simulink model "c00020M_harness"  (R2018a)
settings: Solver=ode3  StartTime=0.0  StopTime=10.0  RelTol=1e-3  EnableMultiTasking=on
undefined symbols (not defined in the file): b, DiscIntNeverNeededParam, J, K, L, PosMinimaW4, R, sigbuilder_block
(part 6 of 41)

== system c00020M_harness/M020 ==
  DW1 : Inport  OutMin=0  OutMax=4  OutDataTypeStr=int8
  DW4 : Inport  Port=2  OutMin=0  OutMax=4  OutDataTypeStr=int8
  P1W2 : Inport  Port=3  OutMin=0  OutMax=4  OutDataTypeStr=int8
  P3W4 : Inport  Port=4  OutMin=0  OutMax=4  OutDataTypeStr=int8
  O1 : Inport  Port=5  OutDataTypeStr=boolean
  O2 : Inport  Port=6  OutDataTypeStr=boolean
  O4 : Inport  Port=7  OutDataTypeStr=boolean
  LD : Inport  Port=8  OutDataTypeStr=boolean
  Cyber : Subsystem
  M : Memory
  M1 : Memory
  M3 : Memory
  Physical : Subsystem
  S1 : Subsystem
  S2 : Subsystem
  S4 : Subsystem
  W1Pos : Outport
  W2Pos : Outport  Port=2
  W4Pos : Outport  Port=3
  wires:
  Cyber/3(W4) -> Physical/3(InW4)
  DW4/1 -> Cyber/5(DW4)
  Physical/3(W4) -> S4/1(PhyMeasure), W4Pos/1
  P3W4/1 -> Cyber/7(P3W4)
  S2/1(SensorOut) -> M1/1
  Physical/2(W2) -> S2/1(PhyMeasure), W2Pos/1
  DW1/1 -> Cyber/4(DW1)
  M/1 -> Cyber/1(PosW1)
  M1/1 -> Cyber/2(PosW2)
  S4/1(SensorOut) -> M3/1
  P1W2/1 -> Cyber/6(P1W2)
  Cyber/2(W2) -> Physical/2(InW2)
  Cyber/1(W1) -> Physical/1(InW1)
  O1/1 -> Cyber/8(OW1)
  LD/1 -> Cyber/11(LD)
  O2/1 -> Cyber/9(OW2)
  O4/1 -> Cyber/10(OW4)
  Physical/1(W1) -> S1/1(PhyMeasure), W1Pos/1
  S1/1(SensorOut) -> M/1
  M3/1 -> Cyber/3(PosW4)

== system c00020M_harness/M022 ==
  DW1 : Inport  OutMin=0  OutMax=4  OutDataTypeStr=int8
  DW4 : Inport  Port=2  OutMin=0  OutMax=4  OutDataTypeStr=int8
  P1W2 : Inport  Port=3  OutMin=0  OutMax=4  OutDataTypeStr=int8
  P3W4 : Inport  Port=4  OutMin=0  OutMax=4  OutDataTypeStr=int8
  O1 : Inport  Port=5  OutDataTypeStr=boolean
  O2 : Inport  Port=6  OutDataTypeStr=boolean
  O4 : Inport  Port=7  OutDataTypeStr=boolean
  LD : Inport  Port=8  OutDataTypeStr=boolean
  Cyber : Subsystem
  M : Memory
  M1 : Memory
  M3 : Memory
  Physical : Subsystem
  S1 : Subsystem
  S2 : Subsystem
  S4 : Subsystem
  W1Pos : Outport
  W2Pos : Outport  Port=2
  W4Pos : Outport  Port=3
  wires:
  Cyber/3(W4) -> Physical/3(InW4)
  DW4/1 -> Cyber/5(DW4)
  Physical/3(W4) -> S4/1(PhyMeasure), W4Pos/1
  P3W4/1 -> Cyber/7(P3W4)
  S2/1(SensorOut) -> M1/1
  Physical/2(W2) -> S2/1(PhyMeasure), W2Pos/1
  DW1/1 -> Cyber/4(DW1)
  M/1 -> Cyber/1(PosW1)
  M1/1 -> Cyber/2(PosW2)
  S4/1(SensorOut) -> M3/1
  P1W2/1 -> Cyber/6(P1W2)
  Cyber/2(W2) -> Physical/2(InW2)
  Cyber/1(W1) -> Physical/1(InW1)
  O1/1 -> Cyber/8(OW1)
  LD/1 -> Cyber/11(LD)
  O2/1 -> Cyber/9(OW2)
  O4/1 -> Cyber/10(OW4)
  Physical/1(W1) -> S1/1(PhyMeasure), W1Pos/1
  S1/1(SensorOut) -> M/1
  M3/1 -> Cyber/3(PosW4)

== system c00020M_harness/M023 ==
  DW1 : Inport  OutMin=0  OutMax=4  OutDataTypeStr=int8
  DW4 : Inport  Port=2  OutMin=0  OutMax=4  OutDataTypeStr=int8
  P1W2 : Inport  Port=3  OutMin=0  OutMax=4  OutDataTypeStr=int8
  P3W4 : Inport  Port=4  OutMin=0  OutMax=4  OutDataTypeStr=int8
  O1 : Inport  Port=5  OutDataTypeStr=boolean
  O2 : Inport  Port=6  OutDataTypeStr=boolean
  O4 : Inport  Port=7  OutDataTypeStr=boolean
  LD : Inport  Port=8  OutDataTypeStr=boolean
  Cyber : Subsystem
  M : Memory
  M1 : Memory
  M3 : Memory
  Physical : Subsystem
  S1 : Subsystem
  S2 : Subsystem
  S4 : Subsystem
  W1Pos : Outport
  W2Pos : Outport  Port=2
  W4Pos : Outport  Port=3
  wires:
  Cyber/3(W4) -> Physical/3(InW4)
  DW4/1 -> Cyber/5(DW4)
  Physical/3(W4) -> S4/1(PhyMeasure), W4Pos/1
  P3W4/1 -> Cyber/7(P3W4)
  S2/1(SensorOut) -> M1/1
  Physical/2(W2) -> S2/1(PhyMeasure), W2Pos/1
  DW1/1 -> Cyber/4(DW1)
  M/1 -> Cyber/1(PosW1)
  M1/1 -> Cyber/2(PosW2)
  S4/1(SensorOut) -> M3/1
  P1W2/1 -> Cyber/6(P1W2)
  Cyber/2(W2) -> Physical/2(InW2)
  Cyber/1(W1) -> Physical/1(InW1)
  O1/1 -> Cyber/8(OW1)
  LD/1 -> Cyber/11(LD)
  O2/1 -> Cyber/9(OW2)
  O4/1 -> Cyber/10(OW4)
  Physical/1(W1) -> S1/1(PhyMeasure), W1Pos/1
  S1/1(SensorOut) -> M/1
  M3/1 -> Cyber/3(PosW4)

== system c00020M_harness/M024 ==
  DW1 : Inport  OutMin=0  OutMax=4  OutDataTypeStr=int8
  DW4 : Inport  Port=2  OutMin=0  OutMax=4  OutDataTypeStr=int8
  P1W2 : Inport  Port=3  OutMin=0  OutMax=4  OutDataTypeStr=int8
  P3W4 : Inport  Port=4  OutMin=0  OutMax=4  OutDataTypeStr=int8
  O1 : Inport  Port=5  OutDataTypeStr=boolean
  O2 : Inport  Port=6  OutDataTypeStr=boolean
  O4 : Inport  Port=7  OutDataTypeStr=boolean
  LD : Inport  Port=8  OutDataTypeStr=boolean
  Cyber : Subsystem
  M : Memory
  M1 : Memory
  M3 : Memory
  Physical : Subsystem
  S1 : Subsystem
  S2 : Subsystem
  S4 : Subsystem
  W1Pos : Outport
  W2Pos : Outport  Port=2
  W4Pos : Outport  Port=3
  wires:
  Cyber/3(W4) -> Physical/3(InW4)
  DW4/1 -> Cyber/5(DW4)
  Physical/3(W4) -> S4/1(PhyMeasure), W4Pos/1
  P3W4/1 -> Cyber/7(P3W4)
  S2/1(SensorOut) -> M1/1
  Physical/2(W2) -> S2/1(PhyMeasure), W2Pos/1
  DW1/1 -> Cyber/4(DW1)
  M/1 -> Cyber/1(PosW1)
  M1/1 -> Cyber/2(PosW2)
  S4/1(SensorOut) -> M3/1
  P1W2/1 -> Cyber/6(P1W2)
  Cyber/2(W2) -> Physical/2(InW2)
  Cyber/1(W1) -> Physical/1(InW1)
  O1/1 -> Cyber/8(OW1)
  LD/1 -> Cyber/11(LD)
  O2/1 -> Cyber/9(OW2)
  O4/1 -> Cyber/10(OW4)
  Physical/1(W1) -> S1/1(PhyMeasure), W1Pos/1
  S1/1(SensorOut) -> M/1
  M3/1 -> Cyber/3(PosW4)

== system c00020M_harness/M026 ==
  DW1 : Inport  OutMin=0  OutMax=4  OutDataTypeStr=int8
  DW4 : Inport  Port=2  OutMin=0  OutMax=4  OutDataTypeStr=int8
  P1W2 : Inport  Port=3  OutMin=0  OutMax=4  OutDataTypeStr=int8
  P3W4 : Inport  Port=4  OutMin=0  OutMax=4  OutDataTypeStr=int8
  O1 : Inport  Port=5  OutDataTypeStr=boolean
  O2 : Inport  Port=6  OutDataTypeStr=boolean
  O4 : Inport  Port=7  OutDataTypeStr=boolean
  LD : Inport  Port=8  OutDataTypeStr=boolean
  Cyber : Subsystem
  M : Memory
  M1 : Memory
  M3 : Memory
  Physical : Subsystem
  S1 : Subsystem
  S2 : Subsystem
  S4 : Subsystem
  W1Pos : Outport
  W2Pos : Outport  Port=2
  W4Pos : Outport  Port=3
  wires:
  Cyber/3(W4) -> Physical/3(InW4)
  DW4/1 -> Cyber/5(DW4)
  Physical/3(W4) -> S4/1(PhyMeasure), W4Pos/1
  P3W4/1 -> Cyber/7(P3W4)
  S2/1(SensorOut) -> M1/1
  Physical/2(W2) -> S2/1(PhyMeasure), W2Pos/1
  DW1/1 -> Cyber/4(DW1)
  M/1 -> Cyber/1(PosW1)
  M1/1 -> Cyber/2(PosW2)
  S4/1(SensorOut) -> M3/1
  P1W2/1 -> Cyber/6(P1W2)
  Cyber/2(W2) -> Physical/2(InW2)
  Cyber/1(W1) -> Physical/1(InW1)
  O1/1 -> Cyber/8(OW1)
  LD/1 -> Cyber/11(LD)
  O2/1 -> Cyber/9(OW2)
  O4/1 -> Cyber/10(OW4)
  Physical/1(W1) -> S1/1(PhyMeasure), W1Pos/1
  S1/1(SensorOut) -> M/1
  M3/1 -> Cyber/3(PosW4)

== system c00020M_harness/M027 ==
  DW1 : Inport  OutMin=0  OutMax=4  OutDataTypeStr=int8
  DW4 : Inport  Port=2  OutMin=0  OutMax=4  OutDataTypeStr=int8
  P1W2 : Inport  Port=3  OutMin=0  OutMax=4  OutDataTypeStr=int8
  P3W4 : Inport  Port=4  OutMin=0  OutMax=4  OutDataTypeStr=int8
  O1 : Inport  Port=5  OutDataTypeStr=boolean
  O2 : Inport  Port=6  OutDataTypeStr=boolean
  O4 : Inport  Port=7  OutDataTypeStr=boolean
  LD : Inport  Port=8  OutDataTypeStr=boolean
  Cyber : Subsystem
  M : Memory
  M1 : Memory
  M3 : Memory
  Physical : Subsystem
  S1 : Subsystem
  S2 : Subsystem
  S4 : Subsystem
  W1Pos : Outport
  W2Pos : Outport  Port=2
  W4Pos : Outport  Port=3
  wires:
  Cyber/3(W4) -> Physical/3(InW4)
  DW4/1 -> Cyber/5(DW4)
  Physical/3(W4) -> S4/1(PhyMeasure), W4Pos/1
  P3W4/1 -> Cyber/7(P3W4)
  S2/1(SensorOut) -> M1/1
  Physical/2(W2) -> S2/1(PhyMeasure), W2Pos/1
  DW1/1 -> Cyber/4(DW1)
  M/1 -> Cyber/1(PosW1)
  M1/1 -> Cyber/2(PosW2)
  S4/1(SensorOut) -> M3/1
  P1W2/1 -> Cyber/6(P1W2)
  Cyber/2(W2) -> Physical/2(InW2)
  Cyber/1(W1) -> Physical/1(InW1)
  O1/1 -> Cyber/8(OW1)
  LD/1 -> Cyber/11(LD)
  O2/1 -> Cyber/9(OW2)
  O4/1 -> Cyber/10(OW4)
  Physical/1(W1) -> S1/1(PhyMeasure), W1Pos/1
  S1/1(SensorOut) -> M/1
  M3/1 -> Cyber/3(PosW4)

== system c00020M_harness/M028 ==
  DW1 : Inport  OutMin=0  OutMax=4  OutDataTypeStr=int8
  DW4 : Inport  Port=2  OutMin=0  OutMax=4  OutDataTypeStr=int8
  P1W2 : Inport  Port=3  OutMin=0  OutMax=4  OutDataTypeStr=int8
  P3W4 : Inport  Port=4  OutMin=0  OutMax=4  OutDataTypeStr=int8
  O1 : Inport  Port=5  OutDataTypeStr=boolean
  O2 : Inport  Port=6  OutDataTypeStr=boolean
  O4 : Inport  Port=7  OutDataTypeStr=boolean
  LD : Inport  Port=8  OutDataTypeStr=boolean
  Cyber : Subsystem
  M : Memory
  M1 : Memory
  M3 : Memory
  Physical : Subsystem
  S1 : Subsystem
  S2 : Subsystem
  S4 : Subsystem
  W1Pos : Outport
  W2Pos : Outport  Port=2
  W4Pos : Outport  Port=3
  wires:
  Cyber/3(W4) -> Physical/3(InW4)
  DW4/1 -> Cyber/5(DW4)
  Physical/3(W4) -> S4/1(PhyMeasure), W4Pos/1
  P3W4/1 -> Cyber/7(P3W4)
  S2/1(SensorOut) -> M1/1
  Physical/2(W2) -> S2/1(PhyMeasure), W2Pos/1
  DW1/1 -> Cyber/4(DW1)
  M/1 -> Cyber/1(PosW1)
  M1/1 -> Cyber/2(PosW2)
  S4/1(SensorOut) -> M3/1
  P1W2/1 -> Cyber/6(P1W2)
  Cyber/2(W2) -> Physical/2(InW2)
  Cyber/1(W1) -> Physical/1(InW1)
  O1/1 -> Cyber/8(OW1)
  LD/1 -> Cyber/11(LD)
  O2/1 -> Cyber/9(OW2)
  O4/1 -> Cyber/10(OW4)
  Physical/1(W1) -> S1/1(PhyMeasure), W1Pos/1
  S1/1(SensorOut) -> M/1
  M3/1 -> Cyber/3(PosW4)

== system c00020M_harness/M030 ==
  DW1 : Inport  OutMin=0  OutMax=4  OutDataTypeStr=int8
  DW4 : Inport  Port=2  OutMin=0  OutMax=4  OutDataTypeStr=int8
  P1W2 : Inport  Port=3  OutMin=0  OutMax=4  OutDataTypeStr=int8
  P3W4 : Inport  Port=4  OutMin=0  OutMax=4  OutDataTypeStr=int8
  O1 : Inport  Port=5  OutDataTypeStr=boolean
  O2 : Inport  Port=6  OutDataTypeStr=boolean
  O4 : Inport  Port=7  OutDataTypeStr=boolean
  LD : Inport  Port=8  OutDataTypeStr=boolean
  Cyber : Subsystem
  M : Memory
  M1 : Memory
  M3 : Memory
  Physical : Subsystem
  S1 : Subsystem
  S2 : Subsystem
  S4 : Subsystem
  W1Pos : Outport
  W2Pos : Outport  Port=2
  W4Pos : Outport  Port=3
  wires:
  Cyber/3(W4) -> Physical/3(InW4)
  DW4/1 -> Cyber/5(DW4)
  Physical/3(W4) -> S4/1(PhyMeasure), W4Pos/1
  P3W4/1 -> Cyber/7(P3W4)
  S2/1(SensorOut) -> M1/1
  Physical/2(W2) -> S2/1(PhyMeasure), W2Pos/1
  DW1/1 -> Cyber/4(DW1)
  M/1 -> Cyber/1(PosW1)
  M1/1 -> Cyber/2(PosW2)
  S4/1(SensorOut) -> M3/1
  P1W2/1 -> Cyber/6(P1W2)
  Cyber/2(W2) -> Physical/2(InW2)
  Cyber/1(W1) -> Physical/1(InW1)
  O1/1 -> Cyber/8(OW1)
  LD/1 -> Cyber/11(LD)
  O2/1 -> Cyber/9(OW2)
  O4/1 -> Cyber/10(OW4)
  Physical/1(W1) -> S1/1(PhyMeasure), W1Pos/1
  S1/1(SensorOut) -> M/1
  M3/1 -> Cyber/3(PosW4)

== system c00020M_harness/M031 ==
  DW1 : Inport  OutMin=0  OutMax=4  OutDataTypeStr=int8
  DW4 : Inport  Port=2  OutMin=0  OutMax=4  OutDataTypeStr=int8
  P1W2 : Inport  Port=3  OutMin=0  OutMax=4  OutDataTypeStr=int8
  P3W4 : Inport  Port=4  OutMin=0  OutMax=4  OutDataTypeStr=int8
  O1 : Inport  Port=5  OutDataTypeStr=boolean
  O2 : Inport  Port=6  OutDataTypeStr=boolean
  O4 : Inport  Port=7  OutDataTypeStr=boolean
  LD : Inport  Port=8  OutDataTypeStr=boolean
  Cyber : Subsystem
  M : Memory
  M1 : Memory
  M3 : Memory
  Physical : Subsystem
  S1 : Subsystem
  S2 : Subsystem
  S4 : Subsystem
  W1Pos : Outport
  W2Pos : Outport  Port=2
  W4Pos : Outport  Port=3
  wires:
  Cyber/3(W4) -> Physical/3(InW4)
  DW4/1 -> Cyber/5(DW4)
  Physical/3(W4) -> S4/1(PhyMeasure), W4Pos/1
  P3W4/1 -> Cyber/7(P3W4)
  S2/1(SensorOut) -> M1/1
  Physical/2(W2) -> S2/1(PhyMeasure), W2Pos/1
  DW1/1 -> Cyber/4(DW1)
  M/1 -> Cyber/1(PosW1)
  M1/1 -> Cyber/2(PosW2)
  S4/1(SensorOut) -> M3/1
  P1W2/1 -> Cyber/6(P1W2)
  Cyber/2(W2) -> Physical/2(InW2)
  Cyber/1(W1) -> Physical/1(InW1)
  O1/1 -> Cyber/8(OW1)
  LD/1 -> Cyber/11(LD)
  O2/1 -> Cyber/9(OW2)
  O4/1 -> Cyber/10(OW4)
  Physical/1(W1) -> S1/1(PhyMeasure), W1Pos/1
  S1/1(SensorOut) -> M/1
  M3/1 -> Cyber/3(PosW4)

== system c00020M_harness/M032 ==
  DW1 : Inport  OutMin=0  OutMax=4  OutDataTypeStr=int8
  DW4 : Inport  Port=2  OutMin=0  OutMax=4  OutDataTypeStr=int8
  P1W2 : Inport  Port=3  OutMin=0  OutMax=4  OutDataTypeStr=int8
  P3W4 : Inport  Port=4  OutMin=0  OutMax=4  OutDataTypeStr=int8
  O1 : Inport  Port=5  OutDataTypeStr=boolean
  O2 : Inport  Port=6  OutDataTypeStr=boolean
  O4 : Inport  Port=7  OutDataTypeStr=boolean
  LD : Inport  Port=8  OutDataTypeStr=boolean
  Cyber : Subsystem
  M : Memory
  M1 : Memory
  M3 : Memory
  Physical : Subsystem
  S1 : Subsystem
  S2 : Subsystem
  S4 : Subsystem
  W1Pos : Outport
  W2Pos : Outport  Port=2
  W4Pos : Outport  Port=3
  wires:
  Cyber/3(W4) -> Physical/3(InW4)
  DW4/1 -> Cyber/5(DW4)
  Physical/3(W4) -> S4/1(PhyMeasure), W4Pos/1
  P3W4/1 -> Cyber/7(P3W4)
  S2/1(SensorOut) -> M1/1
  Physical/2(W2) -> S2/1(PhyMeasure), W2Pos/1
  DW1/1 -> Cyber/4(DW1)
  M/1 -> Cyber/1(PosW1)
  M1/1 -> Cyber/2(PosW2)
  S4/1(SensorOut) -> M3/1
  P1W2/1 -> Cyber/6(P1W2)
  Cyber/2(W2) -> Physical/2(InW2)
  Cyber/1(W1) -> Physical/1(InW1)
  O1/1 -> Cyber/8(OW1)
  LD/1 -> Cyber/11(LD)
  O2/1 -> Cyber/9(OW2)
  O4/1 -> Cyber/10(OW4)
  Physical/1(W1) -> S1/1(PhyMeasure), W1Pos/1
  S1/1(SensorOut) -> M/1
  M3/1 -> Cyber/3(PosW4)

== system c00020M_harness/M034 ==
  DW1 : Inport  OutMin=0  OutMax=4  OutDataTypeStr=int8
  DW4 : Inport  Port=2  OutMin=0  OutMax=4  OutDataTypeStr=int8
  P1W2 : Inport  Port=3  OutMin=0  OutMax=4  OutDataTypeStr=int8
  P3W4 : Inport  Port=4  OutMin=0  OutMax=4  OutDataTypeStr=int8
  O1 : Inport  Port=5  OutDataTypeStr=boolean
  O2 : Inport  Port=6  OutDataTypeStr=boolean
  O4 : Inport  Port=7  OutDataTypeStr=boolean
  LD : Inport  Port=8  OutDataTypeStr=boolean
  Cyber : Subsystem
  M : Memory
  M1 : Memory
  M3 : Memory
  Physical : Subsystem
  S1 : Subsystem
  S2 : Subsystem
  S4 : Subsystem
  W1Pos : Outport
  W2Pos : Outport  Port=2
  W4Pos : Outport  Port=3
  wires:
  Cyber/3(W4) -> Physical/3(InW4)
  DW4/1 -> Cyber/5(DW4)
  Physical/3(W4) -> S4/1(PhyMeasure), W4Pos/1
  P3W4/1 -> Cyber/7(P3W4)
  S2/1(SensorOut) -> M1/1
  Physical/2(W2) -> S2/1(PhyMeasure), W2Pos/1
  DW1/1 -> Cyber/4(DW1)
  M/1 -> Cyber/1(PosW1)
  M1/1 -> Cyber/2(PosW2)
  S4/1(SensorOut) -> M3/1
  P1W2/1 -> Cyber/6(P1W2)
  Cyber/2(W2) -> Physical/2(InW2)
  Cyber/1(W1) -> Physical/1(InW1)
  O1/1 -> Cyber/8(OW1)
  LD/1 -> Cyber/11(LD)
  O2/1 -> Cyber/9(OW2)
  O4/1 -> Cyber/10(OW4)
  Physical/1(W1) -> S1/1(PhyMeasure), W1Pos/1
  S1/1(SensorOut) -> M/1
  M3/1 -> Cyber/3(PosW4)

== system c00020M_harness/M035 ==
  DW1 : Inport  OutMin=0  OutMax=4  OutDataTypeStr=int8
  DW4 : Inport  Port=2  OutMin=0  OutMax=4  OutDataTypeStr=int8
  P1W2 : Inport  Port=3  OutMin=0  OutMax=4  OutDataTypeStr=int8
  P3W4 : Inport  Port=4  OutMin=0  OutMax=4  OutDataTypeStr=int8
  O1 : Inport  Port=5  OutDataTypeStr=boolean
  O2 : Inport  Port=6  OutDataTypeStr=boolean
  O4 : Inport  Port=7  OutDataTypeStr=boolean
  LD : Inport  Port=8  OutDataTypeStr=boolean
  Cyber : Subsystem
  M : Memory
  M1 : Memory
  M3 : Memory
  Physical : Subsystem
  S1 : Subsystem
  S2 : Subsystem
  S4 : Subsystem
  W1Pos : Outport
  W2Pos : Outport  Port=2
  W4Pos : Outport  Port=3
  wires:
  Cyber/3(W4) -> Physical/3(InW4)
  DW4/1 -> Cyber/5(DW4)
  Physical/3(W4) -> S4/1(PhyMeasure), W4Pos/1
  P3W4/1 -> Cyber/7(P3W4)
  S2/1(SensorOut) -> M1/1
  Physical/2(W2) -> S2/1(PhyMeasure), W2Pos/1
  DW1/1 -> Cyber/4(DW1)
  M/1 -> Cyber/1(PosW1)
  M1/1 -> Cyber/2(PosW2)
  S4/1(SensorOut) -> M3/1
  P1W2/1 -> Cyber/6(P1W2)
  Cyber/2(W2) -> Physical/2(InW2)
  Cyber/1(W1) -> Physical/1(InW1)
  O1/1 -> Cyber/8(OW1)
  LD/1 -> Cyber/11(LD)
  O2/1 -> Cyber/9(OW2)
  O4/1 -> Cyber/10(OW4)
  Physical/1(W1) -> S1/1(PhyMeasure), W1Pos/1
  S1/1(SensorOut) -> M/1
  M3/1 -> Cyber/3(PosW4)

== system c00020M_harness/M036 ==
  DW1 : Inport  OutMin=0  OutMax=4  OutDataTypeStr=int8
  DW4 : Inport  Port=2  OutMin=0  OutMax=4  OutDataTypeStr=int8
  P1W2 : Inport  Port=3  OutMin=0  OutMax=4  OutDataTypeStr=int8
  P3W4 : Inport  Port=4  OutMin=0  OutMax=4  OutDataTypeStr=int8
  O1 : Inport  Port=5  OutDataTypeStr=boolean
  O2 : Inport  Port=6  OutDataTypeStr=boolean
  O4 : Inport  Port=7  OutDataTypeStr=boolean
  LD : Inport  Port=8  OutDataTypeStr=boolean
  Cyber : Subsystem
  M : Memory
  M1 : Memory
  M3 : Memory
  Physical : Subsystem
  S1 : Subsystem
  S2 : Subsystem
  S4 : Subsystem
  W1Pos : Outport
  W2Pos : Outport  Port=2
  W4Pos : Outport  Port=3
  wires:
  Cyber/3(W4) -> Physical/3(InW4)
  DW4/1 -> Cyber/5(DW4)
  Physical/3(W4) -> S4/1(PhyMeasure), W4Pos/1
  P3W4/1 -> Cyber/7(P3W4)
  S2/1(SensorOut) -> M1/1
  Physical/2(W2) -> S2/1(PhyMeasure), W2Pos/1
  DW1/1 -> Cyber/4(DW1)
  M/1 -> Cyber/1(PosW1)
  M1/1 -> Cyber/2(PosW2)
  S4/1(SensorOut) -> M3/1
  P1W2/1 -> Cyber/6(P1W2)
  Cyber/2(W2) -> Physical/2(InW2)
  Cyber/1(W1) -> Physical/1(InW1)
  O1/1 -> Cyber/8(OW1)
  LD/1 -> Cyber/11(LD)
  O2/1 -> Cyber/9(OW2)
  O4/1 -> Cyber/10(OW4)
  Physical/1(W1) -> S1/1(PhyMeasure), W1Pos/1
  S1/1(SensorOut) -> M/1
  M3/1 -> Cyber/3(PosW4)

== system c00020M_harness/M038 ==
  DW1 : Inport  OutMin=0  OutMax=4  OutDataTypeStr=int8
  DW4 : Inport  Port=2  OutMin=0  OutMax=4  OutDataTypeStr=int8
  P1W2 : Inport  Port=3  OutMin=0  OutMax=4  OutDataTypeStr=int8
  P3W4 : Inport  Port=4  OutMin=0  OutMax=4  OutDataTypeStr=int8
  O1 : Inport  Port=5  OutDataTypeStr=boolean
  O2 : Inport  Port=6  OutDataTypeStr=boolean
  O4 : Inport  Port=7  OutDataTypeStr=boolean
  LD : Inport  Port=8  OutDataTypeStr=boolean
  Cyber : Subsystem
  M : Memory
  M1 : Memory
  M3 : Memory
  Physical : Subsystem
  S1 : Subsystem
  S2 : Subsystem
  S4 : Subsystem
  W1Pos : Outport
  W2Pos : Outport  Port=2
  W4Pos : Outport  Port=3
  wires:
  Cyber/3(W4) -> Physical/3(InW4)
  DW4/1 -> Cyber/5(DW4)
  Physical/3(W4) -> S4/1(PhyMeasure), W4Pos/1
  P3W4/1 -> Cyber/7(P3W4)
  S2/1(SensorOut) -> M1/1
  Physical/2(W2) -> S2/1(PhyMeasure), W2Pos/1
  DW1/1 -> Cyber/4(DW1)
  M/1 -> Cyber/1(PosW1)
  M1/1 -> Cyber/2(PosW2)
  S4/1(SensorOut) -> M3/1
  P1W2/1 -> Cyber/6(P1W2)
  Cyber/2(W2) -> Physical/2(InW2)
  Cyber/1(W1) -> Physical/1(InW1)
  O1/1 -> Cyber/8(OW1)
  LD/1 -> Cyber/11(LD)
  O2/1 -> Cyber/9(OW2)
  O4/1 -> Cyber/10(OW4)
  Physical/1(W1) -> S1/1(PhyMeasure), W1Pos/1
  S1/1(SensorOut) -> M/1
  M3/1 -> Cyber/3(PosW4)

== system c00020M_harness/M039 ==
  DW1 : Inport  OutMin=0  OutMax=4  OutDataTypeStr=int8
  DW4 : Inport  Port=2  OutMin=0  OutMax=4  OutDataTypeStr=int8
  P1W2 : Inport  Port=3  OutMin=0  OutMax=4  OutDataTypeStr=int8
  P3W4 : Inport  Port=4  OutMin=0  OutMax=4  OutDataTypeStr=int8
  O1 : Inport  Port=5  OutDataTypeStr=boolean
  O2 : Inport  Port=6  OutDataTypeStr=boolean
  O4 : Inport  Port=7  OutDataTypeStr=boolean
  LD : Inport  Port=8  OutDataTypeStr=boolean
  Cyber : Subsystem
  M : Memory
  M1 : Memory
  M3 : Memory
  Physical : Subsystem
  S1 : Subsystem
  S2 : Subsystem
  S4 : Subsystem
  W1Pos : Outport
  W2Pos : Outport  Port=2
  W4Pos : Outport  Port=3
  wires:
  Cyber/3(W4) -> Physical/3(InW4)
  DW4/1 -> Cyber/5(DW4)
  Physical/3(W4) -> S4/1(PhyMeasure), W4Pos/1
  P3W4/1 -> Cyber/7(P3W4)
  S2/1(SensorOut) -> M1/1
  Physical/2(W2) -> S2/1(PhyMeasure), W2Pos/1
  DW1/1 -> Cyber/4(DW1)
  M/1 -> Cyber/1(PosW1)
  M1/1 -> Cyber/2(PosW2)
  S4/1(SensorOut) -> M3/1
  P1W2/1 -> Cyber/6(P1W2)
  Cyber/2(W2) -> Physical/2(InW2)
  Cyber/1(W1) -> Physical/1(InW1)
  O1/1 -> Cyber/8(OW1)
  LD/1 -> Cyber/11(LD)
  O2/1 -> Cyber/9(OW2)
  O4/1 -> Cyber/10(OW4)
  Physical/1(W1) -> S1/1(PhyMeasure), W1Pos/1
  S1/1(SensorOut) -> M/1
  M3/1 -> Cyber/3(PosW4)

== system c00020M_harness/M040 ==
  DW1 : Inport  OutMin=0  OutMax=4  OutDataTypeStr=int8
  DW4 : Inport  Port=2  OutMin=0  OutMax=4  OutDataTypeStr=int8
  P1W2 : Inport  Port=3  OutMin=0  OutMax=4  OutDataTypeStr=int8
  P3W4 : Inport  Port=4  OutMin=0  OutMax=4  OutDataTypeStr=int8
  O1 : Inport  Port=5  OutDataTypeStr=boolean
  O2 : Inport  Port=6  OutDataTypeStr=boolean
  O4 : Inport  Port=7  OutDataTypeStr=boolean
  LD : Inport  Port=8  OutDataTypeStr=boolean
  Cyber : Subsystem
  M : Memory
  M1 : Memory
  M3 : Memory
  Physical : Subsystem
  S1 : Subsystem
  S2 : Subsystem
  S4 : Subsystem
  W1Pos : Outport
  W2Pos : Outport  Port=2
  W4Pos : Outport  Port=3
  wires:
  Cyber/3(W4) -> Physical/3(InW4)
  DW4/1 -> Cyber/5(DW4)
  Physical/3(W4) -> S4/1(PhyMeasure), W4Pos/1
  P3W4/1 -> Cyber/7(P3W4)
  S2/1(SensorOut) -> M1/1
  Physical/2(W2) -> S2/1(PhyMeasure), W2Pos/1
  DW1/1 -> Cyber/4(DW1)
  M/1 -> Cyber/1(PosW1)
  M1/1 -> Cyber/2(PosW2)
  S4/1(SensorOut) -> M3/1
  P1W2/1 -> Cyber/6(P1W2)
  Cyber/2(W2) -> Physical/2(InW2)
  Cyber/1(W1) -> Physical/1(InW1)
  O1/1 -> Cyber/8(OW1)
  LD/1 -> Cyber/11(LD)
  O2/1 -> Cyber/9(OW2)
  O4/1 -> Cyber/10(OW4)
  Physical/1(W1) -> S1/1(PhyMeasure), W1Pos/1
  S1/1(SensorOut) -> M/1
  M3/1 -> Cyber/3(PosW4)

== system c00020M_harness/M042 ==
  DW1 : Inport  OutMin=0  OutMax=4  OutDataTypeStr=int8
  DW4 : Inport  Port=2  OutMin=0  OutMax=4  OutDataTypeStr=int8
  P1W2 : Inport  Port=3  OutMin=0  OutMax=4  OutDataTypeStr=int8
  P3W4 : Inport  Port=4  OutMin=0  OutMax=4  OutDataTypeStr=int8
  O1 : Inport  Port=5  OutDataTypeStr=boolean
  O2 : Inport  Port=6  OutDataTypeStr=boolean
  O4 : Inport  Port=7  OutDataTypeStr=boolean
  LD : Inport  Port=8  OutDataTypeStr=boolean
  Cyber : Subsystem
  M : Memory
  M1 : Memory
  M3 : Memory
  Physical : Subsystem
  S1 : Subsystem
  S2 : Subsystem
  S4 : Subsystem
  W1Pos : Outport
  W2Pos : Outport  Port=2
  W4Pos : Outport  Port=3
  wires:
  Cyber/3(W4) -> Physical/3(InW4)
  DW4/1 -> Cyber/5(DW4)
  Physical/3(W4) -> S4/1(PhyMeasure), W4Pos/1
  P3W4/1 -> Cyber/7(P3W4)
  S2/1(SensorOut) -> M1/1
  Physical/2(W2) -> S2/1(PhyMeasure), W2Pos/1
  DW1/1 -> Cyber/4(DW1)
  M/1 -> Cyber/1(PosW1)
  M1/1 -> Cyber/2(PosW2)
  S4/1(SensorOut) -> M3/1
  P1W2/1 -> Cyber/6(P1W2)
  Cyber/2(W2) -> Physical/2(InW2)
  Cyber/1(W1) -> Physical/1(InW1)
  O1/1 -> Cyber/8(OW1)
  LD/1 -> Cyber/11(LD)
  O2/1 -> Cyber/9(OW2)
  O4/1 -> Cyber/10(OW4)
  Physical/1(W1) -> S1/1(PhyMeasure), W1Pos/1
  S1/1(SensorOut) -> M/1
  M3/1 -> Cyber/3(PosW4)

== system c00020M_harness/M043 ==
  DW1 : Inport  OutMin=0  OutMax=4  OutDataTypeStr=int8
  DW4 : Inport  Port=2  OutMin=0  OutMax=4  OutDataTypeStr=int8
  P1W2 : Inport  Port=3  OutMin=0  OutMax=4  OutDataTypeStr=int8
  P3W4 : Inport  Port=4  OutMin=0  OutMax=4  OutDataTypeStr=int8
  O1 : Inport  Port=5  OutDataTypeStr=boolean
  O2 : Inport  Port=6  OutDataTypeStr=boolean
  O4 : Inport  Port=7  OutDataTypeStr=boolean
  LD : Inport  Port=8  OutDataTypeStr=boolean
  Cyber : Subsystem
  M : Memory
  M1 : Memory
  M3 : Memory
  Physical : Subsystem
  S1 : Subsystem
  S2 : Subsystem
  S4 : Subsystem
  W1Pos : Outport
  W2Pos : Outport  Port=2
  W4Pos : Outport  Port=3
  wires:
  Cyber/3(W4) -> Physical/3(InW4)
  DW4/1 -> Cyber/5(DW4)
  Physical/3(W4) -> S4/1(PhyMeasure), W4Pos/1
  P3W4/1 -> Cyber/7(P3W4)
  S2/1(SensorOut) -> M1/1
  Physical/2(W2) -> S2/1(PhyMeasure), W2Pos/1
  DW1/1 -> Cyber/4(DW1)
  M/1 -> Cyber/1(PosW1)
  M1/1 -> Cyber/2(PosW2)
  S4/1(SensorOut) -> M3/1
  P1W2/1 -> Cyber/6(P1W2)
  Cyber/2(W2) -> Physical/2(InW2)
  Cyber/1(W1) -> Physical/1(InW1)
  O1/1 -> Cyber/8(OW1)
  LD/1 -> Cyber/11(LD)
  O2/1 -> Cyber/9(OW2)
  O4/1 -> Cyber/10(OW4)
  Physical/1(W1) -> S1/1(PhyMeasure), W1Pos/1
  S1/1(SensorOut) -> M/1
  M3/1 -> Cyber/3(PosW4)

== system c00020M_harness/M044 ==
  DW1 : Inport  OutMin=0  OutMax=4  OutDataTypeStr=int8
  DW4 : Inport  Port=2  OutMin=0  OutMax=4  OutDataTypeStr=int8
  P1W2 : Inport  Port=3  OutMin=0  OutMax=4  OutDataTypeStr=int8
  P3W4 : Inport  Port=4  OutMin=0  OutMax=4  OutDataTypeStr=int8
  O1 : Inport  Port=5  OutDataTypeStr=boolean
  O2 : Inport  Port=6  OutDataTypeStr=boolean
  O4 : Inport  Port=7  OutDataTypeStr=boolean
  LD : Inport  Port=8  OutDataTypeStr=boolean
  Cyber : Subsystem
  M : Memory
  M1 : Memory
  M3 : Memory
  Physical : Subsystem
  S1 : Subsystem
  S2 : Subsystem
  S4 : Subsystem
  W1Pos : Outport
  W2Pos : Outport  Port=2
  W4Pos : Outport  Port=3
  wires:
  Cyber/3(W4) -> Physical/3(InW4)
  DW4/1 -> Cyber/5(DW4)
  Physical/3(W4) -> S4/1(PhyMeasure), W4Pos/1
  P3W4/1 -> Cyber/7(P3W4)
  S2/1(SensorOut) -> M1/1
  Physical/2(W2) -> S2/1(PhyMeasure), W2Pos/1
  DW1/1 -> Cyber/4(DW1)
  M/1 -> Cyber/1(PosW1)
  M1/1 -> Cyber/2(PosW2)
  S4/1(SensorOut) -> M3/1
  P1W2/1 -> Cyber/6(P1W2)
  Cyber/2(W2) -> Physical/2(InW2)
  Cyber/1(W1) -> Physical/1(InW1)
  O1/1 -> Cyber/8(OW1)
  LD/1 -> Cyber/11(LD)
  O2/1 -> Cyber/9(OW2)
  O4/1 -> Cyber/10(OW4)
  Physical/1(W1) -> S1/1(PhyMeasure), W1Pos/1
  S1/1(SensorOut) -> M/1
  M3/1 -> Cyber/3(PosW4)

== system c00020M_harness/M046 ==
  DW1 : Inport  OutMin=0  OutMax=4  OutDataTypeStr=int8
  DW4 : Inport  Port=2  OutMin=0  OutMax=4  OutDataTypeStr=int8
  P1W2 : Inport  Port=3  OutMin=0  OutMax=4  OutDataTypeStr=int8
  P3W4 : Inport  Port=4  OutMin=0  OutMax=4  OutDataTypeStr=int8
  O1 : Inport  Port=5  OutDataTypeStr=boolean
  O2 : Inport  Port=6  OutDataTypeStr=boolean
  O4 : Inport  Port=7  OutDataTypeStr=boolean
  LD : Inport  Port=8  OutDataTypeStr=boolean
  Cyber : Subsystem
  M : Memory
  M1 : Memory
  M3 : Memory
  Physical : Subsystem
  S1 : Subsystem
  S2 : Subsystem
  S4 : Subsystem
  W1Pos : Outport
  W2Pos : Outport  Port=2
  W4Pos : Outport  Port=3
  wires:
  Cyber/3(W4) -> Physical/3(InW4)
  DW4/1 -> Cyber/5(DW4)
  Physical/3(W4) -> S4/1(PhyMeasure), W4Pos/1
  P3W4/1 -> Cyber/7(P3W4)
  S2/1(SensorOut) -> M1/1
  Physical/2(W2) -> S2/1(PhyMeasure), W2Pos/1
  DW1/1 -> Cyber/4(DW1)
  M/1 -> Cyber/1(PosW1)
  M1/1 -> Cyber/2(PosW2)
  S4/1(SensorOut) -> M3/1
  P1W2/1 -> Cyber/6(P1W2)
  Cyber/2(W2) -> Physical/2(InW2)
  Cyber/1(W1) -> Physical/1(InW1)
  O1/1 -> Cyber/8(OW1)
  LD/1 -> Cyber/11(LD)
  O2/1 -> Cyber/9(OW2)
  O4/1 -> Cyber/10(OW4)
  Physical/1(W1) -> S1/1(PhyMeasure), W1Pos/1
  S1/1(SensorOut) -> M/1
  M3/1 -> Cyber/3(PosW4)

== system c00020M_harness/M047 ==
  DW1 : Inport  OutMin=0  OutMax=4  OutDataTypeStr=int8
  DW4 : Inport  Port=2  OutMin=0  OutMax=4  OutDataTypeStr=int8
  P1W2 : Inport  Port=3  OutMin=0  OutMax=4  OutDataTypeStr=int8
  P3W4 : Inport  Port=4  OutMin=0  OutMax=4  OutDataTypeStr=int8
  O1 : Inport  Port=5  OutDataTypeStr=boolean
  O2 : Inport  Port=6  OutDataTypeStr=boolean
  O4 : Inport  Port=7  OutDataTypeStr=boolean
  LD : Inport  Port=8  OutDataTypeStr=boolean
  Cyber : Subsystem
  M : Memory
  M1 : Memory
  M3 : Memory
  Physical : Subsystem
  S1 : Subsystem
  S2 : Subsystem
  S4 : Subsystem
  W1Pos : Outport
  W2Pos : Outport  Port=2
  W4Pos : Outport  Port=3
  wires:
  Cyber/3(W4) -> Physical/3(InW4)
  DW4/1 -> Cyber/5(DW4)
  Physical/3(W4) -> S4/1(PhyMeasure), W4Pos/1
  P3W4/1 -> Cyber/7(P3W4)
  S2/1(SensorOut) -> M1/1
  Physical/2(W2) -> S2/1(PhyMeasure), W2Pos/1
  DW1/1 -> Cyber/4(DW1)
  M/1 -> Cyber/1(PosW1)
  M1/1 -> Cyber/2(PosW2)
  S4/1(SensorOut) -> M3/1
  P1W2/1 -> Cyber/6(P1W2)
  Cyber/2(W2) -> Physical/2(InW2)
  Cyber/1(W1) -> Physical/1(InW1)
  O1/1 -> Cyber/8(OW1)
  LD/1 -> Cyber/11(LD)
  O2/1 -> Cyber/9(OW2)
  O4/1 -> Cyber/10(OW4)
  Physical/1(W1) -> S1/1(PhyMeasure), W1Pos/1
  S1/1(SensorOut) -> M/1
  M3/1 -> Cyber/3(PosW4)

== system c00020M_harness/M048 ==
  DW1 : Inport  OutMin=0  OutMax=4  OutDataTypeStr=int8
  DW4 : Inport  Port=2  OutMin=0  OutMax=4  OutDataTypeStr=int8
  P1W2 : Inport  Port=3  OutMin=0  OutMax=4  OutDataTypeStr=int8
  P3W4 : Inport  Port=4  OutMin=0  OutMax=4  OutDataTypeStr=int8
  O1 : Inport  Port=5  OutDataTypeStr=boolean
  O2 : Inport  Port=6  OutDataTypeStr=boolean
  O4 : Inport  Port=7  OutDataTypeStr=boolean
  LD : Inport  Port=8  OutDataTypeStr=boolean
  Cyber : Subsystem
  M : Memory
  M1 : Memory
  M3 : Memory
  Physical : Subsystem
  S1 : Subsystem
  S2 : Subsystem
  S4 : Subsystem
  W1Pos : Outport
  W2Pos : Outport  Port=2
  W4Pos : Outport  Port=3
  wires:
  Cyber/3(W4) -> Physical/3(InW4)
  DW4/1 -> Cyber/5(DW4)
  Physical/3(W4) -> S4/1(PhyMeasure), W4Pos/1
  P3W4/1 -> Cyber/7(P3W4)
  S2/1(SensorOut) -> M1/1
  Physical/2(W2) -> S2/1(PhyMeasure), W2Pos/1
  DW1/1 -> Cyber/4(DW1)
  M/1 -> Cyber/1(PosW1)
  M1/1 -> Cyber/2(PosW2)
  S4/1(SensorOut) -> M3/1
  P1W2/1 -> Cyber/6(P1W2)
  Cyber/2(W2) -> Physical/2(InW2)
  Cyber/1(W1) -> Physical/1(InW1)
  O1/1 -> Cyber/8(OW1)
  LD/1 -> Cyber/11(LD)
  O2/1 -> Cyber/9(OW2)
  O4/1 -> Cyber/10(OW4)
  Physical/1(W1) -> S1/1(PhyMeasure), W1Pos/1
  S1/1(SensorOut) -> M/1
  M3/1 -> Cyber/3(PosW4)

== system c00020M_harness/M050 ==
  DW1 : Inport  OutMin=0  OutMax=4  OutDataTypeStr=int8
  DW4 : Inport  Port=2  OutMin=0  OutMax=4  OutDataTypeStr=int8
  P1W2 : Inport  Port=3  OutMin=0  OutMax=4  OutDataTypeStr=int8
  P3W4 : Inport  Port=4  OutMin=0  OutMax=4  OutDataTypeStr=int8
  O1 : Inport  Port=5  OutDataTypeStr=boolean
  O2 : Inport  Port=6  OutDataTypeStr=boolean
  O4 : Inport  Port=7  OutDataTypeStr=boolean
  LD : Inport  Port=8  OutDataTypeStr=boolean
  Cyber : Subsystem
  M : Memory
  M1 : Memory
  M3 : Memory
  Physical : Subsystem
  S1 : Subsystem
  S2 : Subsystem
  S4 : Subsystem
  W1Pos : Outport
  W2Pos : Outport  Port=2
  W4Pos : Outport  Port=3
  wires:
  Cyber/3(W4) -> Physical/3(InW4)
  DW4/1 -> Cyber/5(DW4)
  Physical/3(W4) -> S4/1(PhyMeasure), W4Pos/1
  P3W4/1 -> Cyber/7(P3W4)
  S2/1(SensorOut) -> M1/1
  Physical/2(W2) -> S2/1(PhyMeasure), W2Pos/1
  DW1/1 -> Cyber/4(DW1)
  M/1 -> Cyber/1(PosW1)
  M1/1 -> Cyber/2(PosW2)
  S4/1(SensorOut) -> M3/1
  P1W2/1 -> Cyber/6(P1W2)
  Cyber/2(W2) -> Physical/2(InW2)
  Cyber/1(W1) -> Physical/1(InW1)
  O1/1 -> Cyber/8(OW1)
  LD/1 -> Cyber/11(LD)
  O2/1 -> Cyber/9(OW2)
  O4/1 -> Cyber/10(OW4)
  Physical/1(W1) -> S1/1(PhyMeasure), W1Pos/1
  S1/1(SensorOut) -> M/1
  M3/1 -> Cyber/3(PosW4)

== system c00020M_harness/M051 ==
  DW1 : Inport  OutMin=0  OutMax=4  OutDataTypeStr=int8
  DW4 : Inport  Port=2  OutMin=0  OutMax=4  OutDataTypeStr=int8
  P1W2 : Inport  Port=3  OutMin=0  OutMax=4  OutDataTypeStr=int8
  P3W4 : Inport  Port=4  OutMin=0  OutMax=4  OutDataTypeStr=int8
  O1 : Inport  Port=5  OutDataTypeStr=boolean
  O2 : Inport  Port=6  OutDataTypeStr=boolean
  O4 : Inport  Port=7  OutDataTypeStr=boolean
  LD : Inport  Port=8  OutDataTypeStr=boolean
  Cyber : Subsystem
  M : Memory
  M1 : Memory
  M3 : Memory
  Physical : Subsystem
  S1 : Subsystem
  S2 : Subsystem
  S4 : Subsystem
  W1Pos : Outport
  W2Pos : Outport  Port=2
  W4Pos : Outport  Port=3
  wires:
  Cyber/3(W4) -> Physical/3(InW4)
  DW4/1 -> Cyber/5(DW4)
  Physical/3(W4) -> S4/1(PhyMeasure), W4Pos/1
  P3W4/1 -> Cyber/7(P3W4)
  S2/1(SensorOut) -> M1/1
  Physical/2(W2) -> S2/1(PhyMeasure), W2Pos/1
  DW1/1 -> Cyber/4(DW1)
  M/1 -> Cyber/1(PosW1)
  M1/1 -> Cyber/2(PosW2)
  S4/1(SensorOut) -> M3/1
  P1W2/1 -> Cyber/6(P1W2)
  Cyber/2(W2) -> Physical/2(InW2)
  Cyber/1(W1) -> Physical/1(InW1)
  O1/1 -> Cyber/8(OW1)
  LD/1 -> Cyber/11(LD)
  O2/1 -> Cyber/9(OW2)
  O4/1 -> Cyber/10(OW4)
  Physical/1(W1) -> S1/1(PhyMeasure), W1Pos/1
  S1/1(SensorOut) -> M/1
  M3/1 -> Cyber/3(PosW4)

== system c00020M_harness/M052 ==
  DW1 : Inport  OutMin=0  OutMax=4  OutDataTypeStr=int8
  DW4 : Inport  Port=2  OutMin=0  OutMax=4  OutDataTypeStr=int8
  P1W2 : Inport  Port=3  OutMin=0  OutMax=4  OutDataTypeStr=int8
  P3W4 : Inport  Port=4  OutMin=0  OutMax=4  OutDataTypeStr=int8
  O1 : Inport  Port=5  OutDataTypeStr=boolean
  O2 : Inport  Port=6  OutDataTypeStr=boolean
  O4 : Inport  Port=7  OutDataTypeStr=boolean
  LD : Inport  Port=8  OutDataTypeStr=boolean
  Cyber : Subsystem
  M : Memory
  M1 : Memory
  M3 : Memory
  Physical : Subsystem
  S1 : Subsystem
  S2 : Subsystem
  S4 : Subsystem
  W1Pos : Outport
  W2Pos : Outport  Port=2
  W4Pos : Outport  Port=3
  wires:
  Cyber/3(W4) -> Physical/3(InW4)
  DW4/1 -> Cyber/5(DW4)
  Physical/3(W4) -> S4/1(PhyMeasure), W4Pos/1
  P3W4/1 -> Cyber/7(P3W4)
  S2/1(SensorOut) -> M1/1
  Physical/2(W2) -> S2/1(PhyMeasure), W2Pos/1
  DW1/1 -> Cyber/4(DW1)
  M/1 -> Cyber/1(PosW1)
  M1/1 -> Cyber/2(PosW2)
  S4/1(SensorOut) -> M3/1
  P1W2/1 -> Cyber/6(P1W2)
  Cyber/2(W2) -> Physical/2(InW2)
  Cyber/1(W1) -> Physical/1(InW1)
  O1/1 -> Cyber/8(OW1)
  LD/1 -> Cyber/11(LD)
  O2/1 -> Cyber/9(OW2)
  O4/1 -> Cyber/10(OW4)
  Physical/1(W1) -> S1/1(PhyMeasure), W1Pos/1
  S1/1(SensorOut) -> M/1
  M3/1 -> Cyber/3(PosW4)

== system c00020M_harness/M054 ==
  DW1 : Inport  OutMin=0  OutMax=4  OutDataTypeStr=int8
  DW4 : Inport  Port=2  OutMin=0  OutMax=4  OutDataTypeStr=int8
  P1W2 : Inport  Port=3  OutMin=0  OutMax=4  OutDataTypeStr=int8
  P3W4 : Inport  Port=4  OutMin=0  OutMax=4  OutDataTypeStr=int8
  O1 : Inport  Port=5  OutDataTypeStr=boolean
  O2 : Inport  Port=6  OutDataTypeStr=boolean
  O4 : Inport  Port=7  OutDataTypeStr=boolean
  LD : Inport  Port=8  OutDataTypeStr=boolean
  Cyber : Subsystem
  M : Memory
  M1 : Memory
  M3 : Memory
  Physical : Subsystem
  S1 : Subsystem
  S2 : Subsystem
  S4 : Subsystem
  W1Pos : Outport
  W2Pos : Outport  Port=2
  W4Pos : Outport  Port=3
  wires:
  Cyber/3(W4) -> Physical/3(InW4)
  DW4/1 -> Cyber/5(DW4)
  Physical/3(W4) -> S4/1(PhyMeasure), W4Pos/1
  P3W4/1 -> Cyber/7(P3W4)
  S2/1(SensorOut) -> M1/1
  Physical/2(W2) -> S2/1(PhyMeasure), W2Pos/1
  DW1/1 -> Cyber/4(DW1)
  M/1 -> Cyber/1(PosW1)
  M1/1 -> Cyber/2(PosW2)
  S4/1(SensorOut) -> M3/1
  P1W2/1 -> Cyber/6(P1W2)
  Cyber/2(W2) -> Physical/2(InW2)
  Cyber/1(W1) -> Physical/1(InW1)
  O1/1 -> Cyber/8(OW1)
  LD/1 -> Cyber/11(LD)
  O2/1 -> Cyber/9(OW2)
  O4/1 -> Cyber/10(OW4)
  Physical/1(W1) -> S1/1(PhyMeasure), W1Pos/1
  S1/1(SensorOut) -> M/1
  M3/1 -> Cyber/3(PosW4)

== system c00020M_harness/M055 ==
  DW1 : Inport  OutMin=0  OutMax=4  OutDataTypeStr=int8
  DW4 : Inport  Port=2  OutMin=0  OutMax=4  OutDataTypeStr=int8
  P1W2 : Inport  Port=3  OutMin=0  OutMax=4  OutDataTypeStr=int8
  P3W4 : Inport  Port=4  OutMin=0  OutMax=4  OutDataTypeStr=int8
  O1 : Inport  Port=5  OutDataTypeStr=boolean
  O2 : Inport  Port=6  OutDataTypeStr=boolean
  O4 : Inport  Port=7  OutDataTypeStr=boolean
  LD : Inport  Port=8  OutDataTypeStr=boolean
  Cyber : Subsystem
  M : Memory
  M1 : Memory
  M3 : Memory
  Physical : Subsystem
  S1 : Subsystem
  S2 : Subsystem
  S4 : Subsystem
  W1Pos : Outport
  W2Pos : Outport  Port=2
  W4Pos : Outport  Port=3
  wires:
  Cyber/3(W4) -> Physical/3(InW4)
  DW4/1 -> Cyber/5(DW4)
  Physical/3(W4) -> S4/1(PhyMeasure), W4Pos/1
  P3W4/1 -> Cyber/7(P3W4)
  S2/1(SensorOut) -> M1/1
  Physical/2(W2) -> S2/1(PhyMeasure), W2Pos/1
  DW1/1 -> Cyber/4(DW1)
  M/1 -> Cyber/1(PosW1)
  M1/1 -> Cyber/2(PosW2)
  S4/1(SensorOut) -> M3/1
  P1W2/1 -> Cyber/6(P1W2)
  Cyber/2(W2) -> Physical/2(InW2)
  Cyber/1(W1) -> Physical/1(InW1)
  O1/1 -> Cyber/8(OW1)
  LD/1 -> Cyber/11(LD)
  O2/1 -> Cyber/9(OW2)
  O4/1 -> Cyber/10(OW4)
  Physical/1(W1) -> S1/1(PhyMeasure), W1Pos/1
  S1/1(SensorOut) -> M/1
  M3/1 -> Cyber/3(PosW4)

== system c00020M_harness/M056 ==
  DW1 : Inport  OutMin=0  OutMax=4  OutDataTypeStr=int8
  DW4 : Inport  Port=2  OutMin=0  OutMax=4  OutDataTypeStr=int8
  P1W2 : Inport  Port=3  OutMin=0  OutMax=4  OutDataTypeStr=int8
  P3W4 : Inport  Port=4  OutMin=0  OutMax=4  OutDataTypeStr=int8
  O1 : Inport  Port=5  OutDataTypeStr=boolean
  O2 : Inport  Port=6  OutDataTypeStr=boolean
  O4 : Inport  Port=7  OutDataTypeStr=boolean
  LD : Inport  Port=8  OutDataTypeStr=boolean
  Cyber : Subsystem
  M : Memory
  M1 : Memory
  M3 : Memory
  Physical : Subsystem
  S1 : Subsystem
  S2 : Subsystem
  S4 : Subsystem
  W1Pos : Outport
  W2Pos : Outport  Port=2
  W4Pos : Outport  Port=3
  wires:
  Cyber/3(W4) -> Physical/3(InW4)
  DW4/1 -> Cyber/5(DW4)
  Physical/3(W4) -> S4/1(PhyMeasure), W4Pos/1
  P3W4/1 -> Cyber/7(P3W4)
  S2/1(SensorOut) -> M1/1
  Physical/2(W2) -> S2/1(PhyMeasure), W2Pos/1
  DW1/1 -> Cyber/4(DW1)
  M/1 -> Cyber/1(PosW1)
  M1/1 -> Cyber/2(PosW2)
  S4/1(SensorOut) -> M3/1
  P1W2/1 -> Cyber/6(P1W2)
  Cyber/2(W2) -> Physical/2(InW2)
  Cyber/1(W1) -> Physical/1(InW1)
  O1/1 -> Cyber/8(OW1)
  LD/1 -> Cyber/11(LD)
  O2/1 -> Cyber/9(OW2)
  O4/1 -> Cyber/10(OW4)
  Physical/1(W1) -> S1/1(PhyMeasure), W1Pos/1
  S1/1(SensorOut) -> M/1
  M3/1 -> Cyber/3(PosW4)

== system c00020M_harness/M058 ==
  DW1 : Inport  OutMin=0  OutMax=4  OutDataTypeStr=int8
  DW4 : Inport  Port=2  OutMin=0  OutMax=4  OutDataTypeStr=int8
  P1W2 : Inport  Port=3  OutMin=0  OutMax=4  OutDataTypeStr=int8
  P3W4 : Inport  Port=4  OutMin=0  OutMax=4  OutDataTypeStr=int8
  O1 : Inport  Port=5  OutDataTypeStr=boolean
  O2 : Inport  Port=6  OutDataTypeStr=boolean
  O4 : Inport  Port=7  OutDataTypeStr=boolean
  LD : Inport  Port=8  OutDataTypeStr=boolean
  Cyber : Subsystem
  M : Memory
  M1 : Memory
  M3 : Memory
  Physical : Subsystem
  S1 : Subsystem
  S2 : Subsystem
  S4 : Subsystem
  W1Pos : Outport
  W2Pos : Outport  Port=2
  W4Pos : Outport  Port=3
  wires:
  Cyber/3(W4) -> Physical/3(InW4)
  DW4/1 -> Cyber/5(DW4)
  Physical/3(W4) -> S4/1(PhyMeasure), W4Pos/1
  P3W4/1 -> Cyber/7(P3W4)
  S2/1(SensorOut) -> M1/1
  Physical/2(W2) -> S2/1(PhyMeasure), W2Pos/1
  DW1/1 -> Cyber/4(DW1)
  M/1 -> Cyber/1(PosW1)
  M1/1 -> Cyber/2(PosW2)
  S4/1(SensorOut) -> M3/1
  P1W2/1 -> Cyber/6(P1W2)
  Cyber/2(W2) -> Physical/2(InW2)
  Cyber/1(W1) -> Physical/1(InW1)
  O1/1 -> Cyber/8(OW1)
  LD/1 -> Cyber/11(LD)
  O2/1 -> Cyber/9(OW2)
  O4/1 -> Cyber/10(OW4)
  Physical/1(W1) -> S1/1(PhyMeasure), W1Pos/1
  S1/1(SensorOut) -> M/1
  M3/1 -> Cyber/3(PosW4)

== system c00020M_harness/M059 ==
  DW1 : Inport  OutMin=0  OutMax=4  OutDataTypeStr=int8
  DW4 : Inport  Port=2  OutMin=0  OutMax=4  OutDataTypeStr=int8
  P1W2 : Inport  Port=3  OutMin=0  OutMax=4  OutDataTypeStr=int8
  P3W4 : Inport  Port=4  OutMin=0  OutMax=4  OutDataTypeStr=int8
  O1 : Inport  Port=5  OutDataTypeStr=boolean
  O2 : Inport  Port=6  OutDataTypeStr=boolean
  O4 : Inport  Port=7  OutDataTypeStr=boolean
  LD : Inport  Port=8  OutDataTypeStr=boolean
  Cyber : Subsystem
  M : Memory
  M1 : Memory
  M3 : Memory
  Physical : Subsystem
  S1 : Subsystem
  S2 : Subsystem
  S4 : Subsystem
  W1Pos : Outport
  W2Pos : Outport  Port=2
  W4Pos : Outport  Port=3
  wires:
  Cyber/3(W4) -> Physical/3(InW4)
  DW4/1 -> Cyber/5(DW4)
  Physical/3(W4) -> S4/1(PhyMeasure), W4Pos/1
  P3W4/1 -> Cyber/7(P3W4)
  S2/1(SensorOut) -> M1/1
  Physical/2(W2) -> S2/1(PhyMeasure), W2Pos/1
  DW1/1 -> Cyber/4(DW1)
  M/1 -> Cyber/1(PosW1)
  M1/1 -> Cyber/2(PosW2)
  S4/1(SensorOut) -> M3/1
  P1W2/1 -> Cyber/6(P1W2)
  Cyber/2(W2) -> Physical/2(InW2)
  Cyber/1(W1) -> Physical/1(InW1)
  O1/1 -> Cyber/8(OW1)
  LD/1 -> Cyber/11(LD)
  O2/1 -> Cyber/9(OW2)
  O4/1 -> Cyber/10(OW4)
  Physical/1(W1) -> S1/1(PhyMeasure), W1Pos/1
  S1/1(SensorOut) -> M/1
  M3/1 -> Cyber/3(PosW4)

== system c00020M_harness/M060 ==
  DW1 : Inport  OutMin=0  OutMax=4  OutDataTypeStr=int8
  DW4 : Inport  Port=2  OutMin=0  OutMax=4  OutDataTypeStr=int8
  P1W2 : Inport  Port=3  OutMin=0  OutMax=4  OutDataTypeStr=int8
  P3W4 : Inport  Port=4  OutMin=0  OutMax=4  OutDataTypeStr=int8
  O1 : Inport  Port=5  OutDataTypeStr=boolean
  O2 : Inport  Port=6  OutDataTypeStr=boolean
  O4 : Inport  Port=7  OutDataTypeStr=boolean
  LD : Inport  Port=8  OutDataTypeStr=boolean
  Cyber : Subsystem
  M : Memory
  M1 : Memory
  M3 : Memory
  Physical : Subsystem
  S1 : Subsystem
  S2 : Subsystem
  S4 : Subsystem
  W1Pos : Outport
  W2Pos : Outport  Port=2
  W4Pos : Outport  Port=3
  wires:
  Cyber/3(W4) -> Physical/3(InW4)
  DW4/1 -> Cyber/5(DW4)
  Physical/3(W4) -> S4/1(PhyMeasure), W4Pos/1
  P3W4/1 -> Cyber/7(P3W4)
  S2/1(SensorOut) -> M1/1
  Physical/2(W2) -> S2/1(PhyMeasure), W2Pos/1
  DW1/1 -> Cyber/4(DW1)
  M/1 -> Cyber/1(PosW1)
  M1/1 -> Cyber/2(PosW2)
  S4/1(SensorOut) -> M3/1
  P1W2/1 -> Cyber/6(P1W2)
  Cyber/2(W2) -> Physical/2(InW2)
  Cyber/1(W1) -> Physical/1(InW1)
  O1/1 -> Cyber/8(OW1)
  LD/1 -> Cyber/11(LD)
  O2/1 -> Cyber/9(OW2)
  O4/1 -> Cyber/10(OW4)
  Physical/1(W1) -> S1/1(PhyMeasure), W1Pos/1
  S1/1(SensorOut) -> M/1
  M3/1 -> Cyber/3(PosW4)

== system c00020M_harness/M062 ==
  DW1 : Inport  OutMin=0  OutMax=4  OutDataTypeStr=int8
  DW4 : Inport  Port=2  OutMin=0  OutMax=4  OutDataTypeStr=int8
  P1W2 : Inport  Port=3  OutMin=0  OutMax=4  OutDataTypeStr=int8
  P3W4 : Inport  Port=4  OutMin=0  OutMax=4  OutDataTypeStr=int8
  O1 : Inport  Port=5  OutDataTypeStr=boolean
  O2 : Inport  Port=6  OutDataTypeStr=boolean
  O4 : Inport  Port=7  OutDataTypeStr=boolean
  LD : Inport  Port=8  OutDataTypeStr=boolean
  Cyber : Subsystem
  M : Memory
  M1 : Memory
  M3 : Memory
  Physical : Subsystem
  S1 : Subsystem
  S2 : Subsystem
  S4 : Subsystem
  W1Pos : Outport
  W2Pos : Outport  Port=2
  W4Pos : Outport  Port=3
  wires:
  Cyber/3(W4) -> Physical/3(InW4)
  DW4/1 -> Cyber/5(DW4)
  Physical/3(W4) -> S4/1(PhyMeasure), W4Pos/1
  P3W4/1 -> Cyber/7(P3W4)
  S2/1(SensorOut) -> M1/1
  Physical/2(W2) -> S2/1(PhyMeasure), W2Pos/1
  DW1/1 -> Cyber/4(DW1)
  M/1 -> Cyber/1(PosW1)
  M1/1 -> Cyber/2(PosW2)
  S4/1(SensorOut) -> M3/1
  P1W2/1 -> Cyber/6(P1W2)
  Cyber/2(W2) -> Physical/2(InW2)
  Cyber/1(W1) -> Physical/1(InW1)
  O1/1 -> Cyber/8(OW1)
  LD/1 -> Cyber/11(LD)
  O2/1 -> Cyber/9(OW2)
  O4/1 -> Cyber/10(OW4)
  Physical/1(W1) -> S1/1(PhyMeasure), W1Pos/1
  S1/1(SensorOut) -> M/1
  M3/1 -> Cyber/3(PosW4)

== system c00020M_harness/M063 ==
  DW1 : Inport  OutMin=0  OutMax=4  OutDataTypeStr=int8
  DW4 : Inport  Port=2  OutMin=0  OutMax=4  OutDataTypeStr=int8
  P1W2 : Inport  Port=3  OutMin=0  OutMax=4  OutDataTypeStr=int8
  P3W4 : Inport  Port=4  OutMin=0  OutMax=4  OutDataTypeStr=int8
  O1 : Inport  Port=5  OutDataTypeStr=boolean
  O2 : Inport  Port=6  OutDataTypeStr=boolean
  O4 : Inport  Port=7  OutDataTypeStr=boolean
  LD : Inport  Port=8  OutDataTypeStr=boolean
  Cyber : Subsystem
  M : Memory
  M1 : Memory
  M3 : Memory
  Physical : Subsystem
  S1 : Subsystem
  S2 : Subsystem
  S4 : Subsystem
  W1Pos : Outport
  W2Pos : Outport  Port=2
  W4Pos : Outport  Port=3
  wires:
  Cyber/3(W4) -> Physical/3(InW4)
  DW4/1 -> Cyber/5(DW4)
  Physical/3(W4) -> S4/1(PhyMeasure), W4Pos/1
  P3W4/1 -> Cyber/7(P3W4)
  S2/1(SensorOut) -> M1/1
  Physical/2(W2) -> S2/1(PhyMeasure), W2Pos/1
  DW1/1 -> Cyber/4(DW1)
  M/1 -> Cyber/1(PosW1)
  M1/1 -> Cyber/2(PosW2)
  S4/1(SensorOut) -> M3/1
  P1W2/1 -> Cyber/6(P1W2)
  Cyber/2(W2) -> Physical/2(InW2)
  Cyber/1(W1) -> Physical/1(InW1)
  O1/1 -> Cyber/8(OW1)
  LD/1 -> Cyber/11(LD)
  O2/1 -> Cyber/9(OW2)
  O4/1 -> Cyber/10(OW4)
  Physical/1(W1) -> S1/1(PhyMeasure), W1Pos/1
  S1/1(SensorOut) -> M/1
  M3/1 -> Cyber/3(PosW4)

== system c00020M_harness/M064 ==
  DW1 : Inport  OutMin=0  OutMax=4  OutDataTypeStr=int8
  DW4 : Inport  Port=2  OutMin=0  OutMax=4  OutDataTypeStr=int8
  P1W2 : Inport  Port=3  OutMin=0  OutMax=4  OutDataTypeStr=int8
  P3W4 : Inport  Port=4  OutMin=0  OutMax=4  OutDataTypeStr=int8
  O1 : Inport  Port=5  OutDataTypeStr=boolean
  O2 : Inport  Port=6  OutDataTypeStr=boolean
  O4 : Inport  Port=7  OutDataTypeStr=boolean
  LD : Inport  Port=8  OutDataTypeStr=boolean
  Cyber : Subsystem
  M : Memory
  M1 : Memory
  M3 : Memory
  Physical : Subsystem
  S1 : Subsystem
  S2 : Subsystem
  S4 : Subsystem
  W1Pos : Outport
  W2Pos : Outport  Port=2
  W4Pos : Outport  Port=3
  wires:
  Cyber/3(W4) -> Physical/3(InW4)
  DW4/1 -> Cyber/5(DW4)
  Physical/3(W4) -> S4/1(PhyMeasure), W4Pos/1
  P3W4/1 -> Cyber/7(P3W4)
  S2/1(SensorOut) -> M1/1
  Physical/2(W2) -> S2/1(PhyMeasure), W2Pos/1
  DW1/1 -> Cyber/4(DW1)
  M/1 -> Cyber/1(PosW1)
  M1/1 -> Cyber/2(PosW2)
  S4/1(SensorOut) -> M3/1
  P1W2/1 -> Cyber/6(P1W2)
  Cyber/2(W2) -> Physical/2(InW2)
  Cyber/1(W1) -> Physical/1(InW1)
  O1/1 -> Cyber/8(OW1)
  LD/1 -> Cyber/11(LD)
  O2/1 -> Cyber/9(OW2)
  O4/1 -> Cyber/10(OW4)
  Physical/1(W1) -> S1/1(PhyMeasure), W1Pos/1
  S1/1(SensorOut) -> M/1
  M3/1 -> Cyber/3(PosW4)

== system c00020M_harness/M066 ==
  DW1 : Inport  OutMin=0  OutMax=4  OutDataTypeStr=int8
  DW4 : Inport  Port=2  OutMin=0  OutMax=4  OutDataTypeStr=int8
  P1W2 : Inport  Port=3  OutMin=0  OutMax=4  OutDataTypeStr=int8
  P3W4 : Inport  Port=4  OutMin=0  OutMax=4  OutDataTypeStr=int8
  O1 : Inport  Port=5  OutDataTypeStr=boolean
  O2 : Inport  Port=6  OutDataTypeStr=boolean
  O4 : Inport  Port=7  OutDataTypeStr=boolean
  LD : Inport  Port=8  OutDataTypeStr=boolean
  Cyber : Subsystem
  M : Memory
  M1 : Memory
  M3 : Memory
  Physical : Subsystem
  S1 : Subsystem
  S2 : Subsystem
  S4 : Subsystem
  W1Pos : Outport
  W2Pos : Outport  Port=2
  W4Pos : Outport  Port=3
  wires:
  Cyber/3(W4) -> Physical/3(InW4)
  DW4/1 -> Cyber/5(DW4)
  Physical/3(W4) -> S4/1(PhyMeasure), W4Pos/1
  P3W4/1 -> Cyber/7(P3W4)
  S2/1(SensorOut) -> M1/1
  Physical/2(W2) -> S2/1(PhyMeasure), W2Pos/1
  DW1/1 -> Cyber/4(DW1)
  M/1 -> Cyber/1(PosW1)
  M1/1 -> Cyber/2(PosW2)
  S4/1(SensorOut) -> M3/1
  P1W2/1 -> Cyber/6(P1W2)
  Cyber/2(W2) -> Physical/2(InW2)
  Cyber/1(W1) -> Physical/1(InW1)
  O1/1 -> Cyber/8(OW1)
  LD/1 -> Cyber/11(LD)
  O2/1 -> Cyber/9(OW2)
  O4/1 -> Cyber/10(OW4)
  Physical/1(W1) -> S1/1(PhyMeasure), W1Pos/1
  S1/1(SensorOut) -> M/1
  M3/1 -> Cyber/3(PosW4)

== system c00020M_harness/M067 ==
  DW1 : Inport  OutMin=0  OutMax=4  OutDataTypeStr=int8
  DW4 : Inport  Port=2  OutMin=0  OutMax=4  OutDataTypeStr=int8
  P1W2 : Inport  Port=3  OutMin=0  OutMax=4  OutDataTypeStr=int8
  P3W4 : Inport  Port=4  OutMin=0  OutMax=4  OutDataTypeStr=int8
  O1 : Inport  Port=5  OutDataTypeStr=boolean
  O2 : Inport  Port=6  OutDataTypeStr=boolean
  O4 : Inport  Port=7  OutDataTypeStr=boolean
  LD : Inport  Port=8  OutDataTypeStr=boolean
  Cyber : Subsystem
  M : Memory
  M1 : Memory
  M3 : Memory
  Physical : Subsystem
  S1 : Subsystem
  S2 : Subsystem
  S4 : Subsystem
  W1Pos : Outport
  W2Pos : Outport  Port=2
  W4Pos : Outport  Port=3
  wires:
  Cyber/3(W4) -> Physical/3(InW4)
  DW4/1 -> Cyber/5(DW4)
  Physical/3(W4) -> S4/1(PhyMeasure), W4Pos/1
  P3W4/1 -> Cyber/7(P3W4)
  S2/1(SensorOut) -> M1/1
  Physical/2(W2) -> S2/1(PhyMeasure), W2Pos/1
  DW1/1 -> Cyber/4(DW1)
  M/1 -> Cyber/1(PosW1)
  M1/1 -> Cyber/2(PosW2)
  S4/1(SensorOut) -> M3/1
  P1W2/1 -> Cyber/6(P1W2)
  Cyber/2(W2) -> Physical/2(InW2)
  Cyber/1(W1) -> Physical/1(InW1)
  O1/1 -> Cyber/8(OW1)
  LD/1 -> Cyber/11(LD)
  O2/1 -> Cyber/9(OW2)
  O4/1 -> Cyber/10(OW4)
  Physical/1(W1) -> S1/1(PhyMeasure), W1Pos/1
  S1/1(SensorOut) -> M/1
  M3/1 -> Cyber/3(PosW4)

== system c00020M_harness/M068 ==
  DW1 : Inport  OutMin=0  OutMax=4  OutDataTypeStr=int8
  DW4 : Inport  Port=2  OutMin=0  OutMax=4  OutDataTypeStr=int8
  P1W2 : Inport  Port=3  OutMin=0  OutMax=4  OutDataTypeStr=int8
  P3W4 : Inport  Port=4  OutMin=0  OutMax=4  OutDataTypeStr=int8
  O1 : Inport  Port=5  OutDataTypeStr=boolean
  O2 : Inport  Port=6  OutDataTypeStr=boolean
  O4 : Inport  Port=7  OutDataTypeStr=boolean
  LD : Inport  Port=8  OutDataTypeStr=boolean
  Cyber : Subsystem
  M : Memory
  M1 : Memory
  M3 : Memory
  Physical : Subsystem
  S1 : Subsystem
  S2 : Subsystem
  S4 : Subsystem
  W1Pos : Outport
  W2Pos : Outport  Port=2
  W4Pos : Outport  Port=3
  wires:
  Cyber/3(W4) -> Physical/3(InW4)
  DW4/1 -> Cyber/5(DW4)
  Physical/3(W4) -> S4/1(PhyMeasure), W4Pos/1
  P3W4/1 -> Cyber/7(P3W4)
  S2/1(SensorOut) -> M1/1
  Physical/2(W2) -> S2/1(PhyMeasure), W2Pos/1
  DW1/1 -> Cyber/4(DW1)
  M/1 -> Cyber/1(PosW1)
  M1/1 -> Cyber/2(PosW2)
  S4/1(SensorOut) -> M3/1
  P1W2/1 -> Cyber/6(P1W2)
  Cyber/2(W2) -> Physical/2(InW2)
  Cyber/1(W1) -> Physical/1(InW1)
  O1/1 -> Cyber/8(OW1)
  LD/1 -> Cyber/11(LD)
  O2/1 -> Cyber/9(OW2)
  O4/1 -> Cyber/10(OW4)
  Physical/1(W1) -> S1/1(PhyMeasure), W1Pos/1
  S1/1(SensorOut) -> M/1
  M3/1 -> Cyber/3(PosW4)

== system c00020M_harness/M070 ==
  DW1 : Inport  OutMin=0  OutMax=4  OutDataTypeStr=int8
  DW4 : Inport  Port=2  OutMin=0  OutMax=4  OutDataTypeStr=int8
  P1W2 : Inport  Port=3  OutMin=0  OutMax=4  OutDataTypeStr=int8
  P3W4 : Inport  Port=4  OutMin=0  OutMax=4  OutDataTypeStr=int8
  O1 : Inport  Port=5  OutDataTypeStr=boolean
  O2 : Inport  Port=6  OutDataTypeStr=boolean
  O4 : Inport  Port=7  OutDataTypeStr=boolean
  LD : Inport  Port=8  OutDataTypeStr=boolean
  Cyber : Subsystem
  M : Memory
  M1 : Memory
  M3 : Memory
  Physical : Subsystem
  S1 : Subsystem
  S2 : Subsystem
  S4 : Subsystem
  W1Pos : Outport
  W2Pos : Outport  Port=2
  W4Pos : Outport  Port=3
  wires:
  Cyber/3(W4) -> Physical/3(InW4)
  DW4/1 -> Cyber/5(DW4)
  Physical/3(W4) -> S4/1(PhyMeasure), W4Pos/1
  P3W4/1 -> Cyber/7(P3W4)
  S2/1(SensorOut) -> M1/1
  Physical/2(W2) -> S2/1(PhyMeasure), W2Pos/1
  DW1/1 -> Cyber/4(DW1)
  M/1 -> Cyber/1(PosW1)
  M1/1 -> Cyber/2(PosW2)
  S4/1(SensorOut) -> M3/1
  P1W2/1 -> Cyber/6(P1W2)
  Cyber/2(W2) -> Physical/2(InW2)
  Cyber/1(W1) -> Physical/1(InW1)
  O1/1 -> Cyber/8(OW1)
  LD/1 -> Cyber/11(LD)
  O2/1 -> Cyber/9(OW2)
  O4/1 -> Cyber/10(OW4)
  Physical/1(W1) -> S1/1(PhyMeasure), W1Pos/1
  S1/1(SensorOut) -> M/1
  M3/1 -> Cyber/3(PosW4)

== system c00020M_harness/M071 ==
  DW1 : Inport  OutMin=0  OutMax=4  OutDataTypeStr=int8
  DW4 : Inport  Port=2  OutMin=0  OutMax=4  OutDataTypeStr=int8
  P1W2 : Inport  Port=3  OutMin=0  OutMax=4  OutDataTypeStr=int8
  P3W4 : Inport  Port=4  OutMin=0  OutMax=4  OutDataTypeStr=int8
  O1 : Inport  Port=5  OutDataTypeStr=boolean
  O2 : Inport  Port=6  OutDataTypeStr=boolean
  O4 : Inport  Port=7  OutDataTypeStr=boolean
  LD : Inport  Port=8  OutDataTypeStr=boolean
  Cyber : Subsystem
  M : Memory
  M1 : Memory
  M3 : Memory
  Physical : Subsystem
  S1 : Subsystem
  S2 : Subsystem
  S4 : Subsystem
  W1Pos : Outport
  W2Pos : Outport  Port=2
  W4Pos : Outport  Port=3
  wires:
  Cyber/3(W4) -> Physical/3(InW4)
  DW4/1 -> Cyber/5(DW4)
  Physical/3(W4) -> S4/1(PhyMeasure), W4Pos/1
  P3W4/1 -> Cyber/7(P3W4)
  S2/1(SensorOut) -> M1/1
  Physical/2(W2) -> S2/1(PhyMeasure), W2Pos/1
  DW1/1 -> Cyber/4(DW1)
  M/1 -> Cyber/1(PosW1)
  M1/1 -> Cyber/2(PosW2)
  S4/1(SensorOut) -> M3/1
  P1W2/1 -> Cyber/6(P1W2)
  Cyber/2(W2) -> Physical/2(InW2)
  Cyber/1(W1) -> Physical/1(InW1)
  O1/1 -> Cyber/8(OW1)
  LD/1 -> Cyber/11(LD)
  O2/1 -> Cyber/9(OW2)
  O4/1 -> Cyber/10(OW4)
  Physical/1(W1) -> S1/1(PhyMeasure), W1Pos/1
  S1/1(SensorOut) -> M/1
  M3/1 -> Cyber/3(PosW4)
